simulink model "bus_combined"  (Simulink 8.0)
settings: Solver=ode45  StartTime=0.0  StopTime=10.0  RelTol=1e-3
settings Model: Creator=massif  LastModifiedBy=massif

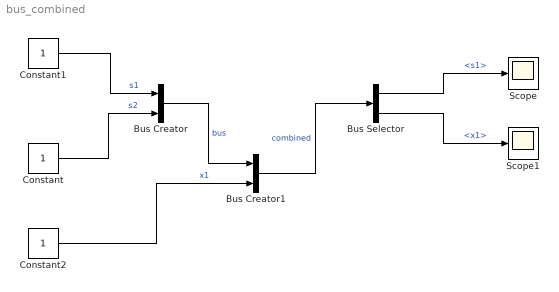
== system bus_combined ==
  Bus Creator : BusCreator  Inputs=2
  Bus Creator1 : BusCreator  Inputs=2
  Bus Selector : BusSelector  OutputSignals=bus.s1,x1
  Constant : Constant
  Constant1 : Constant
  Constant2 : Constant
  Scope : Scope
  Scope1 : Scope
  wires:
  Constant1/1 -> Bus Creator/1  "s1"
  Bus Creator/1 -> Bus Creator1/1  "bus"
  Bus Selector/1 -> Scope/1  "<s1>"
  Bus Selector/2 -> Scope1/1  "<x1>"
  Constant/1 -> Bus Creator/2  "s2"
  Constant2/1 -> Bus Creator1/2  "x1"
  Bus Creator1/1 -> Bus Selector/1  "combined"
